simulink model "sim_variable_structure2"  (R2019a)
settings: Solver=FixedStepAuto  StartTime=0.0  StopTime=end_time  FixedStep=FStep  RelTol=1e-3
undefined symbols (not defined in the file): k1, k2, tau, x0, y0
settings Model: Creator=ogure  LastModifiedBy=ogure
settings SolverCC: SolverResetMethod=Robust
settings DataIOCC: SaveFormat=Array  SaveOutput=off  SignalLogging=off  ReturnWorkspaceOutputs=off
settings DebuggingCC: SolverPrmCheckMsg=warning

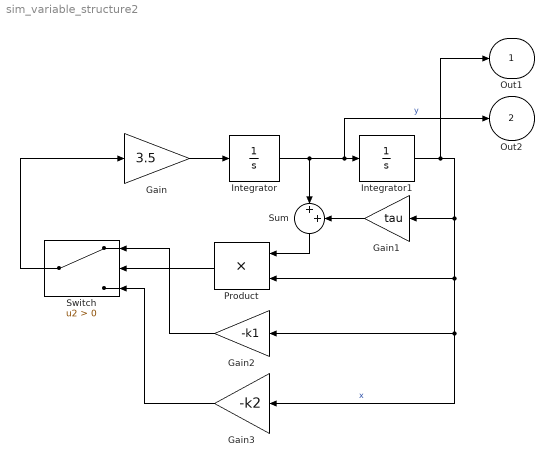
== system sim_variable_structure2 ==
  Gain : Gain  Gain=3.5
  Gain1 : Gain  Gain=tau
  Gain2 : Gain  Gain=-k1
  Gain3 : Gain  Gain=-k2
  Integrator : Integrator  InitialCondition=y0
  Integrator1 : Integrator  InitialCondition=x0
  Product : Product
  Sum : Sum  Inputs=|++
  Switch : Switch  Criteria=u2 > Threshold  ZeroCross=off
  Out1 : Outport  SignalName=x
  Out2 : Outport  Port=2  SignalName=y
  wires:
  Integrator/1 -> Sum/1, Out2/1, Integrator1/1  "y"
  Gain/1 -> Integrator/1
  Product/1 -> Switch/2
  Switch/1 -> Gain/1
  Gain1/1 -> Sum/2
  Integrator1/1 -> Out1/1, Gain3/1, Gain2/1, Product/2, Gain1/1  "x"
  Sum/1 -> Product/1
  Gain2/1 -> Switch/1
  Gain3/1 -> Switch/3
